simulink model "HermiteCubicSplineGeneratorRefMod"  (R2016b)
settings: Solver=VariableStepAuto  StartTime=0.0  StopTime=10.0  RelTol=1e-3
values from neighbouring files (symbols this model uses):
  numberSamplePoints = length(y)    [determineStanceLeg.m]    (also in stance_leg.m)
settings Model: DataDictionary=DataDictionary.sldd  Creator=lucadelaat  LastModifiedBy=Taeke

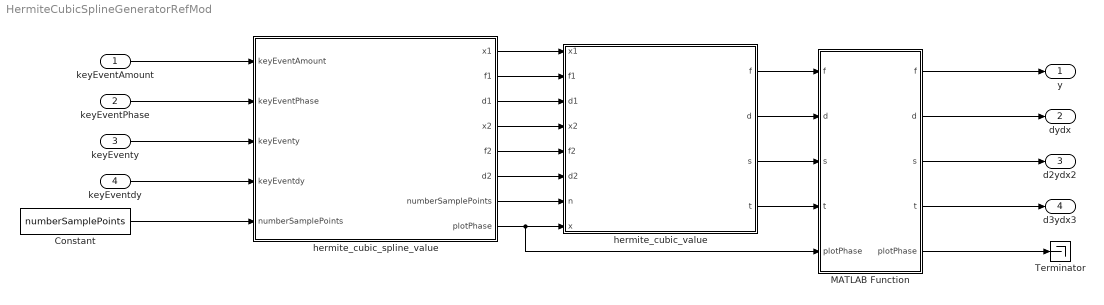
== system HermiteCubicSplineGeneratorRefMod ==
  keyEventAmount : Inport
  keyEventPhase : Inport  Port=2  PortDimensions=keyEventsAmount
  keyEventy : Inport  Port=3  PortDimensions=keyEventsAmount
  keyEventdy : Inport  Port=4  PortDimensions=keyEventsAmount
  Constant : Constant  Value=numberSamplePoints
  MATLAB Function : MATLAB Function  TreatAsAtomicUnit=on
  Terminator : Terminator
  hermite_cubic_spline_value : MATLAB Function  TreatAsAtomicUnit=on
  hermite_cubic_value : MATLAB Function  TreatAsAtomicUnit=on
  y : Outport
  dydx : Outport  Port=2
  d2ydx2 : Outport  Port=3
  d3ydx3 : Outport  Port=4
  wires:
  hermite_cubic_spline_value/1(x1) -> hermite_cubic_value/1(x1)
  hermite_cubic_spline_value/2(f1) -> hermite_cubic_value/2(f1)
  hermite_cubic_spline_value/3(d1) -> hermite_cubic_value/3(d1)
  hermite_cubic_spline_value/4(x2) -> hermite_cubic_value/4(x2)
  hermite_cubic_spline_value/5(f2) -> hermite_cubic_value/5(f2)
  hermite_cubic_spline_value/6(d2) -> hermite_cubic_value/6(d2)
  hermite_cubic_spline_value/7(numberSamplePoints) -> hermite_cubic_value/7(n)
  hermite_cubic_spline_value/8(plotPhase) -> MATLAB Function/5("plotPhase "), hermite_cubic_value/8(x)
  Constant/1 -> hermite_cubic_spline_value/5("numberSamplePoints ")
  keyEventdy/1 -> hermite_cubic_spline_value/4(keyEventdy)
  keyEventy/1 -> hermite_cubic_spline_value/3(keyEventy)
  keyEventPhase/1 -> hermite_cubic_spline_value/2(keyEventPhase)
  keyEventAmount/1 -> hermite_cubic_spline_value/1(keyEventAmount)
  hermite_cubic_value/1(f) -> MATLAB Function/1("f ")
  hermite_cubic_value/2(d) -> MATLAB Function/2("d ")
  hermite_cubic_value/3(s) -> MATLAB Function/3("s ")
  hermite_cubic_value/4(t) -> MATLAB Function/4("t ")
  MATLAB Function/1(f) -> y/1
  MATLAB Function/2(d) -> dydx/1
  MATLAB Function/3(s) -> d2ydx2/1
  MATLAB Function/4(t) -> d3ydx3/1
  MATLAB Function/5(plotPhase) -> Terminator/1

== matlab function HermiteCubicSplineGeneratorRefMod/hermite_cubic_value ==
  data: f output; d output; s output; x1 input; f1 input; d1 input; x2 input; f2 input; d2 input; n input; x input; t output
function [ f, d, s, t ] = hermite_cubic_value( x1, f1, d1, x2, f2, d2, n, x )

%*****************************************************************************80
%
%% HERMITE_CUBIC_VALUE evaluates a Hermite cubic polynomial.
%
%  Discussion:
%
%    The input arguments can be vectors.
%
%  Licensing:
%
%    This code is distributed under the GNU LGPL license.
%
%  Modified:
%
%    12 February 2011
%
%  Author:
%
%    John Burkardt.
%
%  Reference:
%
%    Fred Fritsch, Ralph Carlson,
%    Monotone Piecewise Cubic Interpolation,
%    SIAM Journal on Numerical Analysis,
%    Volume 17, Number 2, April 1980, pages 238-246.
%
%  Parameters:
%
%    Input, real X1, F1, D1, the left endpoint, function value and derivative.
%
%    Input, real X2, F2, D2, the right endpoint, function value and derivative.
%
%    Input, integer N, the number of sample points.
%
%    Input, real X(N), the point at which the Hermite cubic is to be evaluated.
%
%    Output, real F(N), D(N), S(N), T(N), the value and first three derivatives
%    of the Hermite cubic at X.
%
  h =    x2 - x1;
  df = ( f2 - f1 ) ./ h;

  c2 = - ( 2.0 * d1 - 3.0 * df + d2 ) ./ h;
  c3 =   (       d1 - 2.0 * df + d2 ) ./ h ./ h;

  dx = x - x1;
  f = f1 + dx .* ( d1 + dx .* (        c2 + dx .*        c3 ) );
  d =              d1 + dx .* ( 2.0 .* c2 + dx .* 3.0 .* c3 );
  s =                           2.0 .* c2 + dx .* 6.0 .* c3;
  t =                                             6.0 .* c3;

  return
end

== matlab function HermiteCubicSplineGeneratorRefMod/hermite_cubic_spline_value ==
  data: x1 output; f1 output; d1 output; keyEventAmount input; keyEventPhase input; keyEventy input; keyEventdy input; numberSamplePoints input; x2 output; f2 output; d2 output; numberSamplePoints output; plotPhase output
function [ x1, f1, d1, x2, f2, d2, numberSamplePoints, plotPhase ] = hermite_cubic_spline_value( keyEventAmount, keyEventPhase, keyEventy, keyEventdy, numberSamplePoints)

%*****************************************************************************80
%
%% HERMITE_CUBIC_SPLINE_VALUE evaluates a Hermite cubic spline.
%
%  Licensing:
%
%    This code is distributed under the GNU LGPL license.
%
%  Modified:
%
%    27 January 2011
%
%  Author:
%
%    John Burkardt.
%
%  Reference:
%
%    Fred Fritsch, Ralph Carlson,
%    Monotone Piecewise Cubic Interpolation,
%    SIAM Journal on Numerical Analysis,
%    Volume 17, Number 2, April 1980, pages 238-246.
%
%  Parameters:
%
%    Input, integer NN, the number of data points.
%
%    Input, real XN(NN), the coordinates of the data points.
%    The entries in XN must be in strictly ascending order.
%
%    Input, real FN(NN), the function values.
%
%    Input, real DN(NN), the derivative values.
%
%    Input, integer N, the number of sample points.
%
%    Input, real X(N), the coordinates of the sample points.
%
%    Output, real F(N), the function value at the sample points.
%
%    Output, real D(N), the derivative value at the sample points.
%
%    Output, real S(N), the second derivative value at the sample points.
%
%    Output, real T(N), the third derivative value at the sample points.
%

%
%  Remove nan's
%
keyEventPhase = keyEventPhase(~isnan(keyEventPhase));
keyEventy = keyEventy(~isnan(keyEventy));
keyEventdy = keyEventdy(~isnan(keyEventdy));

% Create phase vector
plotPhase = (0:0.1:99.9)';
plotPhase = keyEventPhase(1) + plotPhase;


%
%  Force data to be column vectors.
%

  keyEventPhase = keyEventPhase ( : );
  keyEventy = keyEventy ( : );
  keyEventdy = keyEventdy ( : );
  plotPhase = plotPhase ( : );
%
%  Insert "guard" values of -Inf and +Inf.
%
  xn2 = [ -Inf; keyEventPhase(1:keyEventAmount); +Inf ];
%
%  HISTC returns in I1 the index in XN2 such that
%  XN2(I1(I)) <= X(I) <= XN2(I1(I)+1).
%
  [ n1, i1 ] = histc ( plotPhase, xn2 );
%
%  Assign anything in the (-Inf,XN(1)) bin to (XN(1),XN(2)).
%
  k = find ( i1 == 1 );
  i1(k) = 2;
%
%  Assign anything in the (XN(NN),+Inf) bin to (XN(NN-1),XN(NN)).
%
  k = find ( i1 == keyEventAmount + 1 );
  i1(k) = keyEventAmount;
%
%  Now shift the indices down by 1 because -Inf is fictitious.
%
  i1 = i1 - 1;
%
%  Index the right hand endpoint.
%
  i2 = i1 + 1;

%compute output
  x1 = keyEventPhase(i1);
  f1 = keyEventy(i1);
  d1 = keyEventdy(i1);   
  x2 = keyEventPhase(i2);
  f2 = keyEventy(i2);
  d2 = keyEventdy(i2);
  return
end

== matlab function HermiteCubicSplineGeneratorRefMod/MATLAB Function ==
  data: f input; f output; d input; s input; t input; d output; s output; t output; plotPhase input; plotPhase output
function [f, d, s, t, plotPhase] = fcn(f, d, s, t, plotPhase)

plotPhase = mod(plotPhase,100);

[plotPhase, sortIndex] = sort(plotPhase);
f = f(sortIndex);
d = d(sortIndex);
s = s(sortIndex);
t = t(sortIndex);
end
